simulink library "SwitchStatus"  (R2022a)
settings: Solver=VariableStepAuto  StartTime=0.0  StopTime=10.0  RelTol=1e-3
settings Model: Creator=DELL  LastModifiedBy=DELL

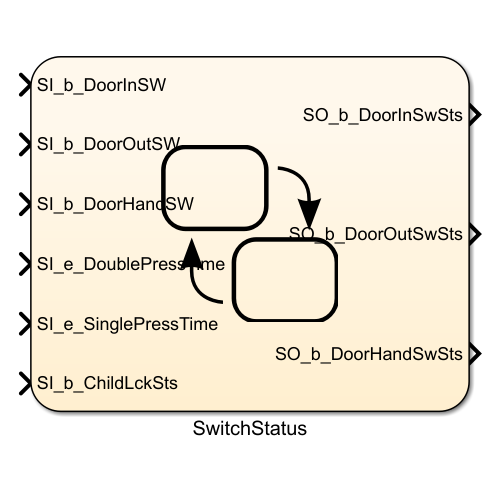
[thumbnail: Simulink's stored preview of the top-level diagram]
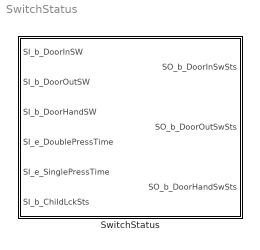
== system SwitchStatus ==
  SwitchStatus : Stateflow chart  TreatAsAtomicUnit=on

== stateflow chart SwitchStatus/SwitchStatus ==
  state DoorInSW [parallel]
    settings: executionOrder=1
    state TWICE
      en:
      SO_b_DoorInSwSts=1;
    state Initial
      en:
      SO_b_DoorInSwSts=0;
    state ONCE
    (default) -> DoorInSW.Initial
    DoorInSW.Initial -> ONCE : [hasChangedTo(SI_b_DoorInSW,1)&&...
        | SI_b_ChildLckSts==0]
    ONCE -> TWICE [order 1] : [hasChangedTo(SI_b_DoorInSW,1)&&...
        | SI_b_ChildLckSts==0]
    ONCE -> DoorInSW.Initial [order 2] : [after(SI_e_DoublePressTime,tick)||...
        | SI_b_ChildLckSts==1]
    TWICE -> DoorInSW.Initial : [after(3,tick)]
  state DoorOutSW [parallel]
    settings: executionOrder=2
    state Initial
      en:
      SO_b_DoorOutSwSts=SI_b_DoorOutSW;
      du:
      SO_b_DoorOutSwSts=SI_b_DoorOutSW;
    (default) -> DoorOutSW.Initial
  state DoorHandSW [parallel]
    settings: executionOrder=3
    state Initial
      en:
      SO_b_DoorHandSwSts=0;
    state Press
    state Release
      en:
      SO_b_DoorHandSwSts=1;
    (default) -> DoorHandSW.Initial
    DoorHandSW.Initial -> Press : [hasChangedTo(SI_b_DoorHandSW,1)]
    Press -> Release [order 1] : [hasChangedTo(SI_b_DoorInSW,0)]
    Press -> DoorHandSW.Initial [order 2] : [after(SI_e_SinglePressTime,tick)]
    Release -> DoorHandSW.Initial : [after(3,tick)]
  data: SI_b_DoorInSW input boolean; SI_b_DoorOutSW input boolean; SI_b_DoorHandSW input boolean; SO_b_DoorInSwSts output boolean; SI_e_DoublePressTime input uint8; SI_e_SinglePressTime input uint8; SI_b_ChildLckSts input boolean; SO_b_DoorOutSwSts output boolean; SO_b_DoorHandSwSts output boolean
